simulink model "SerialSendHF"  (Simulink 9.2)
settings: Solver=FixedStepDiscrete  StartTime=0.0  StopTime=Inf  FixedStep=1/25000  RelTol=1e-3  EnableMultiTasking=on
libraries: simulink x1, c280xlib x1
settings Model: Creator=NRPU  LastModifiedBy=Syed Imtiaz Ali Shah  ExtModeTrigDuration=8
settings Model: SuppressorTable=|
  | <?xml version="1.0" encoding="UTF-8" standalone="yes" ?>
  | <!DOCTYPE boost_serialization>
  | <boost_serialization signature="serialization::archive" version="15">
  | <DiagnosticSuppressor class_id="0" tracking_level="0" version="6">
  | 	<Table class_id="1" tracking_level="0" version="0">
  | 		<count>1</count>
  | 		<bucket_count>8</bucket_count>
  | 		<item_version>0</item_version>
  | 		<item class_id="2" tracking_level="0" version="0">
  | 			<first class_id="3" tracking_level="0" version="6">
  | 				<Source class_id="4" tracking_level="0" version="0">
  | 					<count>1</count>
  | 					<item_version>0</item_version>
  | 					<item>SerialSendHF/Serial Send1/Counter Limited</item>
  | 				</Source>
  | 			</first>
  | 			<second class_id="5" tracking_level="0" version="6">
  | 				<SuppressedData class_id="6" tracking_level="0" version="0">
  | 					<count>2</count>
  | 					<bucket_count>8</bucket_count>
  | 					<item_version>0</item_version>
  | 					<item class_id="7" tracking_level="0" version="0">
  | 						<first class_id="8" tracking_level="0" version="6">
  | 							<ID>SimulinkFixedPoint:util:Overflowoccurred</ID>
  | 							<Cause>
  | 								<Source>
  | 									<count>0</count>
  | 									<item_version>0</item_version>
  | 								</Source>
  | 							</Cause>
  | 						</first>
  | 						<second class_id="9" tracking_level="0" version="6">
  | 							<Comment></Comment>
  | 							<User></User>
  | 							<LastModified class_id="10" tracking_level="0" version="0">
  | 								<ptime_date class_id="11" tracking_level="0" version="0">
  | 									<date>20160608</date>
  | 								</ptime_date>
  | 								<ptime_time_duration class_id="12" tracking_level="0" version="0">
  | 									<is_special>0</is_special>
  | 									<time_duration_hours>15</time_duration_hours>
  | 									<time_duration_minutes>23</time_duration_minutes>
  | 									<time_duration_seconds>17</time_duration_seconds>
  | 									<time_duration_fractional_seconds>0</time_duration_fractional_seconds>
  | 								</ptime_time_duration>
  | 							</LastModified>
  | 							<SuppressionType>1</SuppressionType>
  | 						</second>
  | 					</item>
  | 					<item>
  | 						<first>
  | 							<ID>Simulink:DataType:WarningOverFlowDetected</ID>
  | 							<Cause>
  | 								<Source>
  | 									<count>0</count>
  | 									<item_version>0</item_version>
  | 								</Source>
  | 							</Cause>
  | 						</first>
  | 						<second>
  | 							<Comment></Comment>
  | 							<User></User>
  | 							<LastModified>
  | 								<ptime_date>
  | 									<date>20160608</date>
  | 								</ptime_date>
  | 								<ptime_time_duration>
  | 									<is_special>0</is_special>
  | 									<time_duration_hours>15</time_duration_hours>
  | 									<time_duration_minutes>23</time_duration_minutes>
  | 									<time_duration_seconds>17</time_duration_seconds>
  | 									<time_duration_fractional_seconds>0</time_duration_fractional_seconds>
  | 								</ptime_time_duration>
  | 							</LastModified>
  | 							<SuppressionType>1</SuppressionType>
  | 						</second>
  | 					</item>
  | 				</SuppressedData>
  | 			</second>
  | 		</item>
  | 	</Table>
  | </DiagnosticSuppressor>
  | </boost_serialization>
settings DataIOCC: LimitDataPoints=off  SaveFormat=Dataset  SignalLoggingSaveFormat=Dataset  ReturnWorkspaceOutputs=on
settings OptimizationCC: DefaultUnderspecifiedDataType=single  EnhancedBackFolding=on  PassReuseOutputArgsAs=Individual arguments  LifeSpan=auto  MaxStackSize=512  OptimizeBlockOrder=speed  DifferentSizesBufferReuse=on  OptimizationCustomize=off
settings DebuggingCC: UnderspecifiedInitializationDetection=Simplified  MergeDetectMultiDrivingBlocksExec=error  ParameterTunabilityLossMsg=error  FcnCallInpInsideContextMsg=error  StateNameClashWarn=none  SFUnexpectedBacktrackingDiag=error  SFNoUnconditionalDefaultTransitionDiag=error  SFExecutionAtInitializationDiag=warning  SFMachineParentedDataDiag=error
settings HardwareCC: ProdBitPerChar=16  ProdBitPerInt=16  ProdLargestAtomicInteger=Integer  ProdIntDivRoundTo=Zero  ProdEndianess=LittleEndian  ProdWordSize=16  ProdLongLongMode=on  ProdHWDeviceType=Texas Instruments->C2000
settings ModelReferenceCC: PropagateSignalLabelsOutOfModel=on
settings SFSimCC: SimUseLocalCustomCode=on  MATLABDynamicMemAlloc=off
settings RTWCC: SystemTargetFile=ert.tlc  HardwareBoard=TI Delfino F28379D LaunchPad  TLCOptions=-aInlineSetEventsForThisBaseRateFcn=TLC_FALSE -aSuppressMultiTaskScheduler=TLC_FALSE -aRateBasedStepFcn=1  TemplateMakefile=ert_default_tmf  Description=Embedded Coder  GenerateReport=on  RTWUseLocalCustomCode=on  Toolchain=Texas Instruments Code Composer Studio (C2000)  IncludeHyperlinkInReport=on  LaunchReport=on  GenerateTraceInfo=on  GenerateTraceReport=on  GenerateTraceReportSl=on  GenerateTraceReportSf=on  GenerateTraceReportEml=on
settings MATStruct: className=codertarget.tools.BuildHook  argsTopModelOnly=[]  excludedModels=[]  includeReferencedModels=on  includeTopModel=on  enabled=on  UseCoderTarget=[1]  TargetHardware=TI Delfino F28379D LaunchPad  RTOS=Baremetal  Scheduler_interrupt_source=[0.0]  ExtModeCOMPort=COM6  ExecutionProfileBufferLen=[50.0]  DataVersion=2016.02  IPAddress=codertarget.registry.getLoopbackIP;  Port=17725  Verbose=[0]  Configuration=serial  BuildAction=Build, load and run  DeviceID=F28379D  FlashLoad=[1.0]  CPU=CPU1  LoadCommandArg=$(TARGET_ROOT)/CCS_Config/f28379D.ccxml  CPU2ModelEnable=false  PF1DMAAccess=[0.0]  PF2DMAAccess=[0.0]  UseCustomLinker=[0.0]  cpuClockRateMHz=200  UseInternalOsc=[0.0]  OSCCLK=10  AutoSetPllSettings=[1.0]  PLLCR=40  DIVSEL=2  ClosestCpuClock=200  LspclkDiv=SYSCLKOUT/1  LSPCLK=200  CpuCore=Auto  ClockDiv=SYSCLKOUT/5.0  ClockFrequency=[40.0]  OffsetCorrectionValue=AdcaRegs.ADCOFFTRIM.bit.OFFTRIM  ExternalReferenceSelector=[0.0]  ExternalReferenceVREFHI=3.3  ExternalReferenceVREFLO=0  INTPulseGeneration=Late interrupt pulse  SOCpriority=All in round robin mode  XINT2GPIO=GPIO0  voltage=ADC reference voltage (VREFHIA)  loadmode=System clock (SYSCLK)  PinAssignment_TZ1=None  PinAssignment_TZ2=None  PinAssignment_TZ3=None  PinAssignment_SYNCI=None  PinAssignment_SYNCO=None  PinAssignment_PWM1A=GPIO0  PinAssignment_PWM1B=GPIO1  PinAssignment_PWM2A=GPIO2  PinAssignment_PWM2B=GPIO3  PinAssignment_PWM3A=GPIO4  PinAssignment_PWM3B=GPIO5  PinAssignment_PWM4A=GPIO6  PinAssignment_PWM4B=GPIO7  PinAssignment_PWM5A=GPIO8  PinAssignment_PWM5B=GPIO9  PinAssignment_PWM6A=GPIO10  PinAssignment_PWM6B=GPIO11  PinAssignment_PWM7A=GPIO157  PinAssignment_PWM7B=GPIO158  PinAssignment_PWM8A=GPIO159  PinAssignment_PWM8B=GPIO160  PinAssignment_PWM9A=GPIO16  PinAssignment_PWM9B=GPIO17  PinAssignment_PWM10A=GPIO18  PinAssignment_PWM10B=GPIO19  PinAssignment_PWM11A=GPIO20  PinAssignment_PWM11B=GPIO21  PinAssignment_PWM12A=GPIO22  PinAssignment_PWM12B=GPIO23  PinAssignment_ECAP1=GPIO20  PinAssignment_ECAP2=GPIO21  PinAssignment_ECAP3=GPIO99  PinAssignment_ECAP4=GPIO54  PinAssignment_ECAP5=GPIO55  PinAssignment_ECAP6=GPIO57  PinAssignment_APWM1=GPIO24  PinAssignment_APWM2=GPIO25  PinAssignment_APWM3=GPIO26  PinAssignment_APWM4=GPIO27  PinAssignment_APWM5=GPIO28  PinAssignment_APWM6=GPIO29  PinAssignment_eQEP1A=GPIO20  PinAssignment_eQEP1B=GPIO21  PinAssignment_eQEP1S=None  PinAssignment_eQEP1I=GPIO99  PinAssignment_eQEP2A=GPIO54  PinAssignment_eQEP2B=GPIO55  PinAssignment_eQEP2S=None  PinAssignment_eQEP2I=GPIO57  PinAssignment_eQEP3A=GPIO28  PinAssignment_eQEP3B=GPIO29  PinAssignment_eQEP3S=GPIO30  PinAssignment_eQEP3I=GPIO31  Mode=Master  AddrDataFormat=7-Bit Addressing  OwnAddress=1  BitCount=8  ModuleClockPrescaler=9  ModuleClockFrequency=[20000000.0]  MasterClkLowTime=20  MasterClkHighTime=20  MasterClockFrequency=[400000.0]  MasterClockFrequency_1=[400000.0]  MasterClockFrequency_2=[400000.0]  EnableLoopback=[0.0]  PinAssignment_SDAA=GPIO104  PinAssignment_SCLA=GPIO105  EnableTxInt=[0.0]  TxFifoLevel=0  EnableRxInt=[0.0]  RxFifoLevel=0  EnableSysInt=[0.0]  AAS=[0.0]  SCD=[0.0]  ARDY=[0.0]  NACK=[0.0]  AL=[0.0]  EnableLoopBack=[0.0]  SuspensionMode=Free_run  NumberOfStopBits=1  ParityMode=None  CharacterLengthBits=8  UserBaudRate=12e6  BaudRatePrescaler=[1.0]  BaudRate=[12500000.0]  CommunicationMode=Raw_data  BlockingMode=[0.0]  DataByteOrder=Little_Endian  DataSwapWidth=8_bits  PinAssignment_Tx=GPIO42  PinAssignment_Rx=GPIO43  BaudRateFactor=[108.0]  DataBits=16  ClockPolarity=Rising_edge  ClockPhase=No_delay  EnableThreeWire=[0.0]  TXINTERRUPTENABLE=[0.0]  FIFOInterruptLevel_Tx=0  RXINTERRUPTENABLE=[0.0]  FIFOInterruptLevel_Rx=16  FIFOEnable=[1.0]  FIFOTransmitDelay=0  PinAssignment_SIMO=GPIO58  PinAssignment_SOMI=GPIO59  PinAssignment_CLK=GPIO60  PinAssignment_STE=GPIO61  PinValue_SIMO=58  PinValue_SOMI=59  PinValue_CLK=60  PinValue_STE=61  PinMux_SIMO=15  PinMux_SOMI=15  PinMux_CLK=15  PinMux_STE=15  FIFO_Level=[16.0]  TSEG1=5  TSEG2=4  SBG=Only_falling_edges  SJW=2  SAM=Sample_one_time  EnhancedCANMode=[1.0]  SelfTestMode=[0.0]  Enable_watchdog=[0.0]  Watchdogclock=OSCCLK/512/1  Time_period=[0.0131072]  Watchdogevent=Chip reset  GPIOQualSel0=Synchronize to SYSCLKOUT only  GPIOQualSel1=Synchronize to SYSCLKOUT only  GPIOQualSel2=Synchronize to SYSCLKOUT only  GPIOQualSel3=Synchronize to SYSCLKOUT only  GPIOQualSel4=Synchronize to SYSCLKOUT only  GPIOQualSel5=Synchronize to SYSCLKOUT only  GPIOQualSel6=Synchronize to SYSCLKOUT only  GPIOQualSel7=Synchronize to SYSCLKOUT only  QualPRD=0  GPIOQualSel8=Synchronize to SYSCLKOUT only  GPIOQualSel9=Synchronize to SYSCLKOUT only  GPIOQualSel10=Synchronize to SYSCLKOUT only  GPIOQualSel11=Synchronize to SYSCLKOUT only  GPIOQualSel12=Synchronize to SYSCLKOUT only  GPIOQualSel13=Synchronize to SYSCLKOUT only  GPIOQualSel14=Synchronize to SYSCLKOUT only  GPIOQualSel15=Synchronize to SYSCLKOUT only  GPIOQualSel16=Synchronize to SYSCLKOUT only  GPIOQualSel17=Synchronize to SYSCLKOUT only  GPIOQualSel18=Synchronize to SYSCLKOUT only  GPIOQualSel19=Synchronize to SYSCLKOUT only  GPIOQualSel20=Synchronize to SYSCLKOUT only  GPIOQualSel21=Synchronize to SYSCLKOUT only  GPIOQualSel22=Synchronize to SYSCLKOUT only  GPIOQualSel23=Synchronize to SYSCLKOUT only  GPIOQualSel24=Synchronize to SYSCLKOUT only  GPIOQualSel25=Synchronize to SYSCLKOUT only  GPIOQualSel26=Synchronize to SYSCLKOUT only  GPIOQualSel27=Synchronize to SYSCLKOUT only  GPIOQualSel28=Synchronize to SYSCLKOUT only  GPIOQualSel29=Synchronize to SYSCLKOUT only  GPIOQualSel30=Synchronize to SYSCLKOUT only  GPIOQualSel31=Synchronize to SYSCLKOUT only  GPIOQualSel32=Synchronize to SYSCLKOUT only  GPIOQualSel33=Synchronize to SYSCLKOUT only  GPIOQualSel34=Synchronize to SYSCLKOUT only  GPIOQualSel35=Synchronize to SYSCLKOUT only  GPIOQualSel36=Synchronize to SYSCLKOUT only  GPIOQualSel37=Synchronize to SYSCLKOUT only  GPIOQualSel38=Synchronize to SYSCLKOUT only  GPIOQualSel39=Synchronize to SYSCLKOUT only  GPIOQualSel40=Synchronize to SYSCLKOUT only  GPIOQualSel41=Synchronize to SYSCLKOUT only  GPIOQualSel42=Synchronize to SYSCLKOUT only  GPIOQualSel43=Synchronize to SYSCLKOUT only  GPIOQualSel44=Synchronize to SYSCLKOUT only  GPIOQualSel45=Synchronize to SYSCLKOUT only  GPIOQualSel46=Synchronize to SYSCLKOUT only  GPIOQualSel47=Synchronize to SYSCLKOUT only  GPIOQualSel48=Synchronize to SYSCLKOUT only  GPIOQualSel49=Synchronize to SYSCLKOUT only  GPIOQualSel50=Synchronize to SYSCLKOUT only  GPIOQualSel51=Synchronize to SYSCLKOUT only  GPIOQualSel52=Synchronize to SYSCLKOUT only  GPIOQualSel53=Synchronize to SYSCLKOUT only  GPIOQualSel54=Synchronize to SYSCLKOUT only  GPIOQualSel55=Synchronize to SYSCLKOUT only  GPIOQualSel56=Synchronize to SYSCLKOUT only  GPIOQualSel57=Synchronize to SYSCLKOUT only  GPIOQualSel58=Synchronize to SYSCLKOUT only  GPIOQualSel59=Synchronize to SYSCLKOUT only  GPIOQualSel60=Synchronize to SYSCLKOUT only  GPIOQualSel61=Synchronize to SYSCLKOUT only  GPIOQualSel62=Synchronize to SYSCLKOUT only  GPIOQualSel63=Synchronize to SYSCLKOUT only  GPIOQualSel64=Synchronize to SYSCLKOUT only  GPIOQualSel65=Synchronize to SYSCLKOUT only  GPIOQualSel66=Synchronize to SYSCLKOUT only  GPIOQualSel67=Synchronize to SYSCLKOUT only  GPIOQualSel68=Synchronize to SYSCLKOUT only  GPIOQualSel69=Synchronize to SYSCLKOUT only  GPIOQualSel70=Synchronize to SYSCLKOUT only  GPIOQualSel71=Synchronize to SYSCLKOUT only  GPIOQualSel72=Synchronize to SYSCLKOUT only  GPIOQualSel73=Synchronize to SYSCLKOUT only  GPIOQualSel74=Synchronize to SYSCLKOUT only  GPIOQualSel75=Synchronize to SYSCLKOUT only  GPIOQualSel76=Synchronize to SYSCLKOUT only  GPIOQualSel77=Synchronize to SYSCLKOUT only  GPIOQualSel78=Synchronize to SYSCLKOUT only  GPIOQualSel79=Synchronize to SYSCLKOUT only  GPIOQualSel80=Synchronize to SYSCLKOUT only  GPIOQualSel81=Synchronize to SYSCLKOUT only  GPIOQualSel82=Synchronize to SYSCLKOUT only  GPIOQualSel83=Synchronize to SYSCLKOUT only  GPIOQualSel84=Synchronize to SYSCLKOUT only  GPIOQualSel85=Synchronize to SYSCLKOUT only  GPIOQualSel86=Synchronize to SYSCLKOUT only  GPIOQualSel87=Synchronize to SYSCLKOUT only  GPIOQualSel88=Synchronize to SYSCLKOUT only  GPIOQualSel89=Synchronize to SYSCLKOUT only  GPIOQualSel90=Synchronize to SYSCLKOUT only  GPIOQualSel91=Synchronize to SYSCLKOUT only  GPIOQualSel92=Synchronize to SYSCLKOUT only  GPIOQualSel93=Synchronize to SYSCLKOUT only  GPIOQualSel94=Synchronize to SYSCLKOUT only  GPIOQualSel95=Synchronize to SYSCLKOUT only  GPIOQualSel96=Synchronize to SYSCLKOUT only  GPIOQualSel97=Synchronize to SYSCLKOUT only  GPIOQualSel98=Synchronize to SYSCLKOUT only  GPIOQualSel99=Synchronize to SYSCLKOUT only  GPIOQualSel100=Synchronize to SYSCLKOUT only  GPIOQualSel101=Synchronize to SYSCLKOUT only  GPIOQualSel102=Synchronize to SYSCLKOUT only  GPIOQualSel103=Synchronize to SYSCLKOUT only  GPIOQualSel104=Synchronize to SYSCLKOUT only  GPIOQualSel105=Synchronize to SYSCLKOUT only  GPIOQualSel106=Synchronize to SYSCLKOUT only  GPIOQualSel107=Synchronize to SYSCLKOUT only  GPIOQualSel108=Synchronize to SYSCLKOUT only  GPIOQualSel109=Synchronize to SYSCLKOUT only  GPIOQualSel110=Synchronize to SYSCLKOUT only  GPIOQualSel111=Synchronize to SYSCLKOUT only  GPIOQualSel112=Synchronize to SYSCLKOUT only  GPIOQualSel113=Synchronize to SYSCLKOUT only  GPIOQualSel114=Synchronize to SYSCLKOUT only  GPIOQualSel115=Synchronize to SYSCLKOUT only  GPIOQualSel116=Synchronize to SYSCLKOUT only  GPIOQualSel117=Synchronize to SYSCLKOUT only  GPIOQualSel118=Synchronize to SYSCLKOUT only  GPIOQualSel119=Synchronize to SYSCLKOUT only  GPIOQualSel120=Synchronize to SYSCLKOUT only  GPIOQualSel121=Synchronize to SYSCLKOUT only  GPIOQualSel122=Synchronize to SYSCLKOUT only  GPIOQualSel123=Synchronize to SYSCLKOUT only  GPIOQualSel124=Synchronize to SYSCLKOUT only  GPIOQualSel125=Synchronize to SYSCLKOUT only  GPIOQualSel126=Synchronize to SYSCLKOUT only  GPIOQualSel127=Synchronize to SYSCLKOUT only  GPIOQualSel128=Synchronize to SYSCLKOUT only  GPIOQualSel129=Synchronize to SYSCLKOUT only  GPIOQualSel130=Synchronize to SYSCLKOUT only  GPIOQualSel131=Synchronize to SYSCLKOUT only  GPIOQualSel132=Synchronize to SYSCLKOUT only  GPIOQualSel133=Synchronize to SYSCLKOUT only  GPIOQualSel134=Synchronize to SYSCLKOUT only  GPIOQualSel135=Synchronize to SYSCLKOUT only  GPIOQualSel136=Synchronize to SYSCLKOUT only  GPIOQualSel137=Synchronize to SYSCLKOUT only  GPIOQualSel138=Synchronize to SYSCLKOUT only  GPIOQualSel139=Synchronize to SYSCLKOUT only  GPIOQualSel140=Synchronize to SYSCLKOUT only  GPIOQualSel141=Synchronize to SYSCLKOUT only  GPIOQualSel142=Synchronize to SYSCLKOUT only  GPIOQualSel143=Synchronize to SYSCLKOUT only  GPIOQualSel144=Synchronize to SYSCLKOUT only  GPIOQualSel145=Synchronize to SYSCLKOUT only  GPIOQualSel146=Synchronize to SYSCLKOUT only  GPIOQualSel147=Synchronize to SYSCLKOUT only  GPIOQualSel148=Synchronize to SYSCLKOUT only  GPIOQualSel149=Synchronize to SYSCLKOUT only  GPIOQualSel150=Synchronize to SYSCLKOUT only  GPIOQualSel151=Synchronize to SYSCLKOUT only  GPIOQualSel152=Synchronize to SYSCLKOUT only  GPIOQualSel153=Synchronize to SYSCLKOUT only  GPIOQualSel154=Synchronize to SYSCLKOUT only  GPIOQualSel155=Synchronize to SYSCLKOUT only  GPIOQualSel156=Synchronize to SYSCLKOUT only  GPIOQualSel157=Synchronize to SYSCLKOUT only  GPIOQualSel158=Synchronize to SYSCLKOUT only  GPIOQualSel159=Synchronize to SYSCLKOUT only  GPIOQualSel160=Synchronize to SYSCLKOUT only  GPIOQualSel161=Synchronize to SYSCLKOUT only  GPIOQualSel162=Synchronize to SYSCLKOUT only  GPIOQualSel163=Synchronize to SYSCLKOUT only  GPIOQualSel164=Synchronize to SYSCLKOUT only  GPIOQualSel165=Synchronize to SYSCLKOUT only  GPIOQualSel166=Synchronize to SYSCLKOUT only  GPIOQualSel167=Synchronize to SYSCLKOUT only  GPIOQualSel168=Synchronize to SYSCLKOUT only  GPIOQualSel169=Synchronize to SYSCLKOUT only  GPIOQualSel170=Synchronize to SYSCLKOUT only  GPIOQualSel171=Synchronize to SYSCLKOUT only  GPIOQualSel172=Synchronize to SYSCLKOUT only  GPIOQualSel173=Synchronize to SYSCLKOUT only  GPIOQualSel174=Synchronize to SYSCLKOUT only  GPIOQualSel175=Synchronize to SYSCLKOUT only  EnableDMAChannel=[0.0]  DataSize=16 bit  InterruptSrc=None  BurstSize=1  TransferSize=1  SrcBeginAdd=0xC000  DstBeginAdd=0xD000  SrcBurstStep=0  DstBurstStep=0  SrcTransStep=0  DstTransStep=0  WrapSrcSize=65536  WrapDstSize=65536  SrcWrapStep=0  DstWrapStep=0  SetCh1ToHigh=[0.0]  EnableOneShot=[0.0]  EnableContinuous=[1.0]  GenInterrupt=Never  EnableOverFlow=[0.0]  GPIOXINT1SEL=0  GPIOXINT2SEL=0  GPIOXINT3SEL=0  GPIOXINT4SEL=0  GPIOXINT5SEL=0  Polarity1=Falling edge  Polarity2=Falling edge  Polarity3=Falling edge  Polarity4=Falling edge  Polarity5=Falling edge
settings CodeAppCC: ForceParamTrailComments=on  IgnoreCustomStorageClasses=off  OperatorAnnotations=on  SimulinkDataObjDesc=on  SFDataObjDesc=on  InsertBlockDesc=on  StateflowObjectComments=off
settings ERTTargetCC: CodeReplacementLibrary=TI C28x
settings ConfigComp: CovMetricSettings=dwe  CovHtmlReporting=off  CovSaveCumulativeToWorkspaceVar=off  CovSaveSingleToWorkspaceVar=off  CovExternalEMLEnable=on

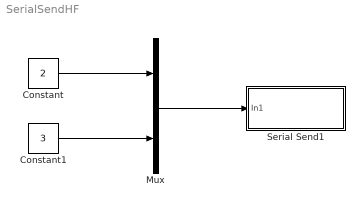
== system SerialSendHF ==
  Constant : Constant  Value=2  OutDataTypeStr=uint16
  Constant1 : Constant  Value=3  OutDataTypeStr=uint16
  Mux : Mux  Inputs=2
  Serial Send1 : Subsystem
  wires:
  Mux/1 -> Serial Send1/1(In1)
  Constant/1 -> Mux/1
  Constant1/1 -> Mux/2

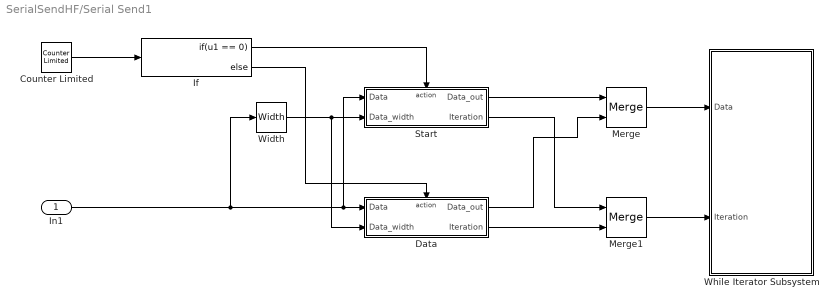
== system SerialSendHF/Serial Send1 ==
  In1 : Inport
  Counter Limited : simulink/Sources/Counter Limited  uplimit=11999  tsamp=-1
  Data : Subsystem  TreatAsAtomicUnit=on
  If : If  IfExpression=u1 == 0
  Merge : Merge
  Merge1 : Merge
  Start : Subsystem  TreatAsAtomicUnit=on
  While Iterator Subsystem : Subsystem  TreatAsAtomicUnit=on
  Width : Width  OutDataTypeMode=All ports same datatype  DataType=uint16
  wires:
  If/1 -> Start/Action
  If/2 -> Data/Action
  Counter Limited/1 -> If/1
  Start/1(Data_out) -> Merge/1
  Data/1(Data_out) -> Merge/2
  Merge/1 -> While Iterator Subsystem/1(Data)
  Merge1/1 -> While Iterator Subsystem/2(Iteration)
  Start/2(Iteration) -> Merge1/1
  Data/2(Iteration) -> Merge1/2
  Width/1 -> Data/2(Data_width), Start/2(Data_width)
  In1/1 -> Width/1, Start/1(Data), Data/1(Data)

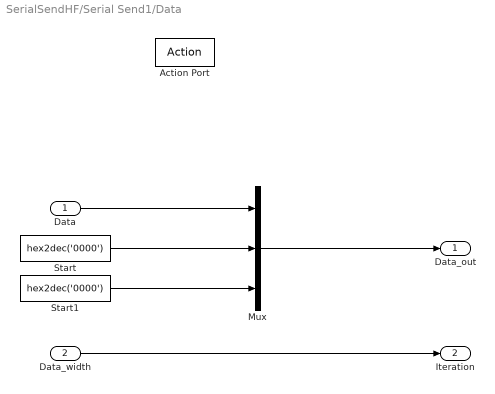
== system SerialSendHF/Serial Send1/Data ==
  Data : Inport
  Data_width : Inport  Port=2
  Action Port : ActionPort  ActionType=else
  Mux : Mux  Inputs=3
  Start : Constant  Value=hex2dec('0000')  OutDataTypeStr=uint16
  Start1 : Constant  Value=hex2dec('0000')  OutDataTypeStr=uint16
  Data_out : Outport
  Iteration : Outport  Port=2
  wires:
  Start/1 -> Mux/2
  Mux/1 -> Data_out/1
  Data/1 -> Mux/1
  Data_width/1 -> Iteration/1
  Start1/1 -> Mux/3

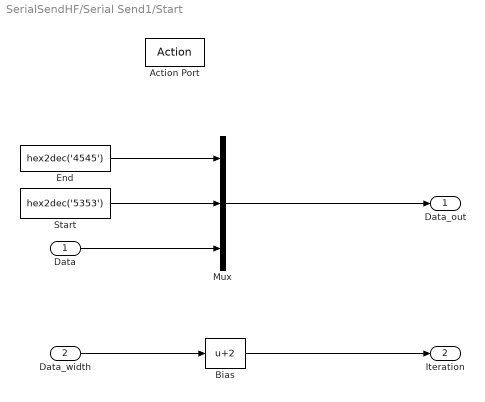
== system SerialSendHF/Serial Send1/Start ==
  Data : Inport
  Data_width : Inport  Port=2
  Action Port : ActionPort  ActionType=then
  Bias : Bias  Bias=2
  End : Constant  Value=hex2dec('4545')  OutDataTypeStr=uint16
  Mux : Mux  Inputs=3
  Start : Constant  Value=hex2dec('5353')  OutDataTypeStr=uint16
  Data_out : Outport
  Iteration : Outport  Port=2
  wires:
  Start/1 -> Mux/2
  Mux/1 -> Data_out/1
  Data_width/1 -> Bias/1
  Bias/1 -> Iteration/1
  Data/1 -> Mux/3
  End/1 -> Mux/1

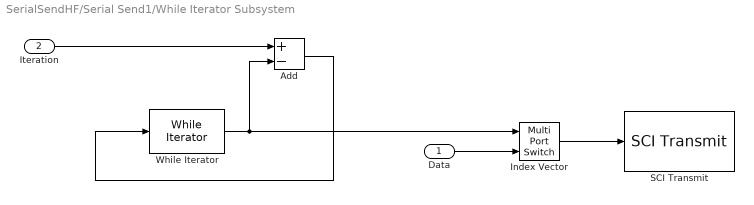
== system SerialSendHF/Serial Send1/While Iterator Subsystem ==
  Data : Inport
  Iteration : Inport  Port=2
  Add : Sum  Inputs=+-  OutDataTypeStr=Inherit: Same as first input
  Index Vector : MultiPortSwitch  Inputs=1
  SCI Transmit : c280xlib/SCI Transmit  sciModule=A  dataHead=''  dataTail=''  postInterrupt=off  numFifo=1
  While Iterator : WhileIterator  MaxIters=-1  WhileBlockType=do-while  ShowIterationPort=on  OutputDataType=int16
  wires:
  Iteration/1 -> Add/1
  Add/1 -> While Iterator/1
  Index Vector/1 -> SCI Transmit/1
  Data/1 -> Index Vector/2
  While Iterator/1 -> Index Vector/1, Add/2
